simulink model "transferfunctionz"  (R2020a)
settings: Solver=VariableStepAuto  StartTime=0.0  StopTime=10.0  RelTol=1e-3
values from neighbouring files (symbols this model uses):
  K_z = 0.1070    (= 0.107)    [Parameters.m]    (also in model_sweep.m = 2)
  kD_z = 13    [Parameters.m]    (also in Untitled6.m = kD_z+i; descent2.m = 13.65; gradient_descent.m = 0.31426857; init.m = 0.3143)
  kP_z = 75    [Parameters.m]    (also in descent2.m = 80; gradient_descent.m = 1.17648234; init.m = 1.1766; model_sweep.m = 40)
  T_aero = 0.2776    [Parameters.m]    (also in model_sweep.m = 2.5)
  T_motor = 0.0640    (= 0.064)    [Parameters.m]
  tau_z = 0.0656    [Parameters.m]
settings Model: Creator=anees  LastModifiedBy=anees

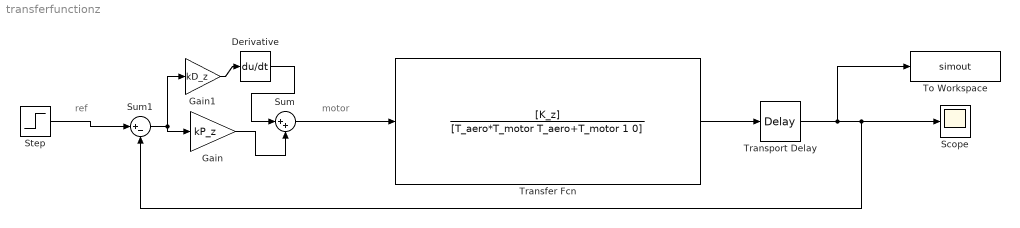
== system transferfunctionz ==
  note: ref
  note: motor
  Derivative : Derivative
  Gain : Gain  Gain=kP_z
  Gain1 : Gain  Gain=kD_z
  Scope : Scope
  Step : Step  SampleTime=0
  Sum : Sum  Inputs=|++
  Sum1 : Sum  Inputs=|+-
  To Workspace : ToWorkspace  VariableName=simout  SaveFormat=Timeseries  SampleTime=-1
  Transfer Fcn : TransferFcn  Numerator=[K_z]  Denominator=[T_aero*T_motor T_aero+T_motor 1 0]
  Transport Delay : TransportDelay  DelayTime=tau_z
  wires:
  Sum/1 -> Transfer Fcn/1
  Transfer Fcn/1 -> Transport Delay/1
  Transport Delay/1 -> To Workspace/1, Scope/1, Sum1/2
  Sum1/1 -> Gain1/1, Gain/1
  Gain1/1 -> Derivative/1
  Derivative/1 -> Sum/1
  Gain/1 -> Sum/2
  Step/1 -> Sum1/1
